simulink model "state_space"  (R2025a)
settings: Solver=VariableStepAuto  StartTime=0.0  StopTime=3  RelTol=1e-3
values from neighbouring files (symbols this model uses):
  A = [-6 -25; 1 0]    [IntPlot.m]
  B = [25; 0]    [IntPlot.m]
  C = [1 0 ; 0 1]    [IntPlot.m]
  D = [0; 0]    [IntPlot.m]
settings Model: Creator=Alex_  LastModifiedBy=Alex_

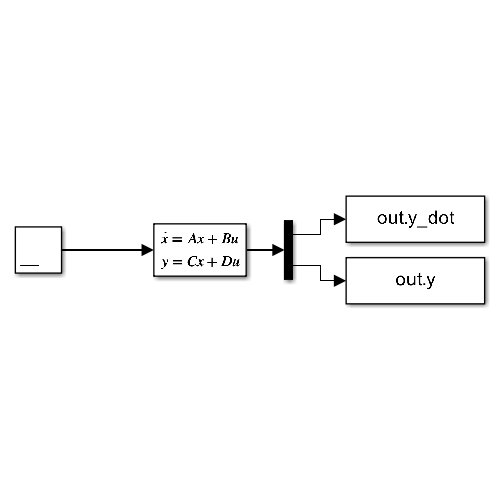
[thumbnail: Simulink's stored preview of the top-level diagram]
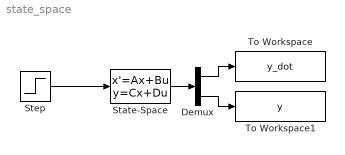
== system state_space ==
  Demux : Demux  Outputs=2
  State-Space : StateSpace  A=A  B=B  C=C  D=D  InitialCondition=0
  Step : Step  Time=0  SampleTime=0
  To Workspace : ToWorkspace  VariableName=y_dot  SampleTime=-1
  To Workspace1 : ToWorkspace  VariableName=y  SampleTime=-1
  wires:
  State-Space/1 -> Demux/1
  Step/1 -> State-Space/1
  Demux/1 -> To Workspace/1
  Demux/2 -> To Workspace1/1
